simulink model "inertialDynamicsTestHarness"  (R2024a)
settings: configuration reference "standardSILConfiguraitonParams" (kept outside this file)
undefined symbols (not defined in the file): aircraftInitialEuler_rad, aircraftInitialPosInNED_m, aircraftInitialVelInBody_mps
settings Model: Creator=jerem  LastModifiedBy=jerem
settings ConfigSetRef: SourceName=standardSILConfiguraitonParams  SourceLocation=Base Workspace

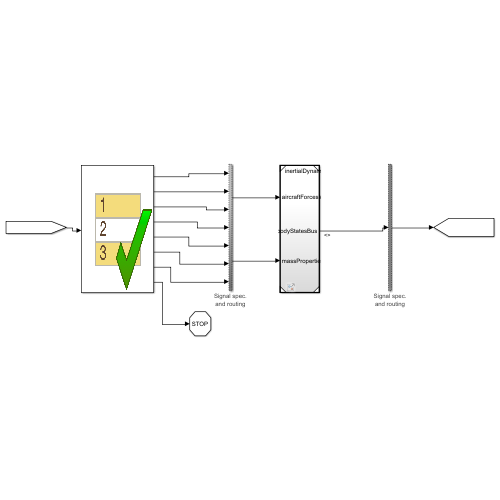
[thumbnail: Simulink's stored preview of the top-level diagram]
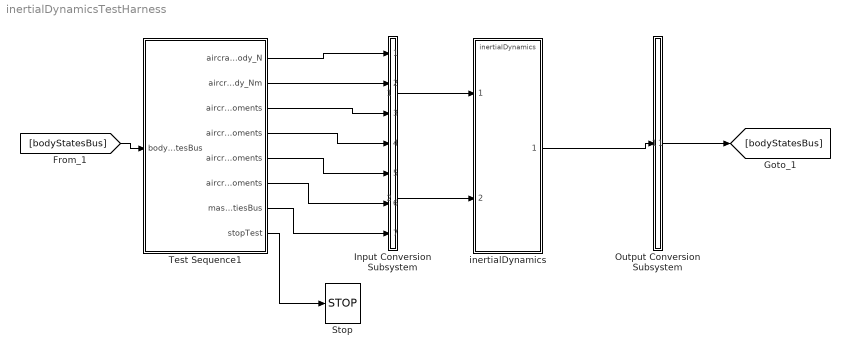
== system inertialDynamicsTestHarness ==
  Input Conversion Subsystem : Subsystem  Tag=__SLT_ICS__  Description=|
      | Signal spec.
      | and routing
      settings: AttributesFormatString=%<Description>
  Output Conversion Subsystem : Subsystem  Tag=__SLT_OCS__  Description=|
      | Signal spec.
      | and routing
      mask init:
      | ICDictionary = get_param(bdroot, 'DataDictionary');
      | if isempty(ICDictionary)
      |    ICScope = Simulink.data.BaseWorkspace;
      | else
      |    ICScope = Simulink.data.DataDictionary(ICDictionary);
      | end
      | 
      | IC1 = Simulink.Bus.createMATLABStruct('BodyStateBus', [], [1 1], ICScope);
      settings: AttributesFormatString=%<Description>
  Stop : Stop
  Test Sequence1 : Test Sequence  TreatAsAtomicUnit=on
  inertialDynamics : ModelReference  ModelNameDialog=inertialDynamics  SimulationMode=Normal  ModelReferenceVersion=1.34
  wires:
  Test Sequence1/1(aircraftForcesMomentsBus_forcesInBody_N) -> Input Conversion Subsystem/1(Inport_1)
  Test Sequence1/2(aircraftForcesMomentsBus_momentsInBody_Nm) -> Input Conversion Subsystem/2(Inport_2)
  Test Sequence1/3(aircraftForcesMomentsBus_aeroForcesMoments) -> Input Conversion Subsystem/3(Inport_3)
  Test Sequence1/4(aircraftForcesMomentsBus_engineForcesMoments) -> Input Conversion Subsystem/4(Inport_4)
  Test Sequence1/5(aircraftForcesMomentsBus_groundForcesMoments) -> Input Conversion Subsystem/5(Inport_5)
  Test Sequence1/6(aircraftForcesMomentsBus_weightForcesMoments) -> Input Conversion Subsystem/6(Inport_6)
  Test Sequence1/7(massPropertiesBus) -> Input Conversion Subsystem/7(Inport_7)
  [bodyStatesBus] -> Test Sequence1/1(bodyStatesBus)
  Output Conversion Subsystem/1(Outport_1) -> [bodyStatesBus]
  Test Sequence1/8(stopTest) -> Stop/1
  inertialDynamics/1 -> Output Conversion Subsystem/1(Inport_1)
  Input Conversion Subsystem/1(Outport_1) -> inertialDynamics/1
  Input Conversion Subsystem/2(Outport_2) -> inertialDynamics/2

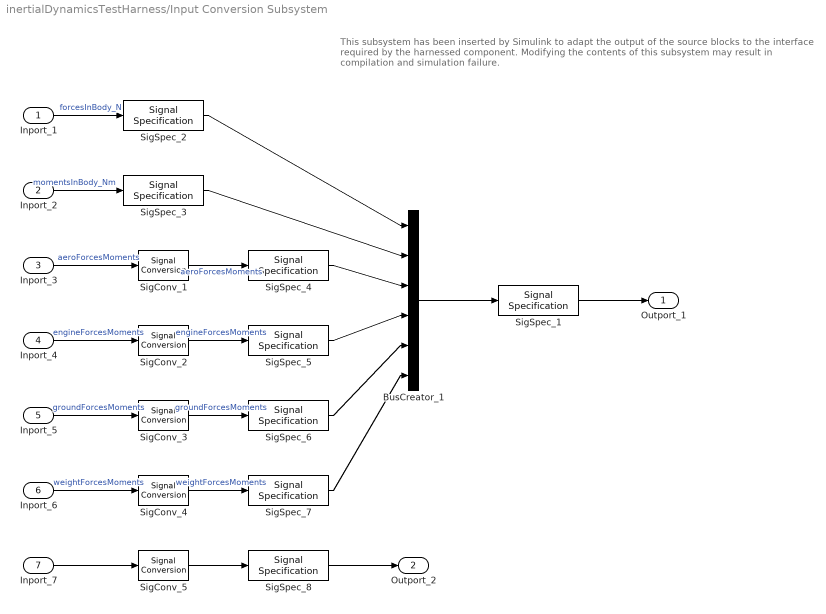
== system inertialDynamicsTestHarness/Input Conversion Subsystem ==
  note: This subsystem has been inserted by Simulink to adapt the output of the source blocks to the interface required by the harnessed component.
      |  Modifying the contents of this subsystem may result in compilation and simulation failure.
  Inport_1 : Inport
  Inport_2 : Inport  Port=2
  Inport_3 : Inport  Port=3
  Inport_4 : Inport  Port=4
  Inport_5 : Inport  Port=5
  Inport_6 : Inport  Port=6
  Inport_7 : Inport  Port=7
  BusCreator_1 : BusCreator  Inputs=6  OutDataTypeStr=Bus: AircraftForcesMomentsBus
  SigConv_{1..4} (4 alike) : SignalConversion  ConversionOutput=Nonvirtual bus  OverrideOpt=off
  SigConv_5 : SignalConversion  ConversionOutput=Virtual bus  OverrideOpt=off
  SigSpec_1 : SignalSpecification  OutDataTypeStr=Bus: AircraftForcesMomentsBus  SampleTime=[-1, 0]
  SigSpec_2 : SignalSpecification  OutDataTypeStr=double  Dimensions=[3]  SampleTime=[-1, 0]
  SigSpec_3 : SignalSpecification  OutDataTypeStr=double  Dimensions=[3]  SampleTime=[-1, 0]
  SigSpec_{4..7} (4 alike) : SignalSpecification  OutDataTypeStr=Bus: ComponentForcesMomentsBus  Dimensions=[1]  SampleTime=[-1, 0]  BusOutputAsStruct=on
  SigSpec_8 : SignalSpecification  OutDataTypeStr=Bus: MassPropertiesBus  SampleTime=[-1, 0]
  Outport_1 : Outport
  Outport_2 : Outport  Port=2
  wires:
  SigSpec_1/1 -> Outport_1/1
  BusCreator_1/1 -> SigSpec_1/1
  SigSpec_2/1 -> BusCreator_1/1
  Inport_1/1 -> SigSpec_2/1  "forcesInBody_N"
  SigSpec_3/1 -> BusCreator_1/2
  Inport_2/1 -> SigSpec_3/1  "momentsInBody_Nm"
  SigSpec_4/1 -> BusCreator_1/3
  SigConv_1/1 -> SigSpec_4/1  "aeroForcesMoments"
  Inport_3/1 -> SigConv_1/1  "aeroForcesMoments"
  SigSpec_5/1 -> BusCreator_1/4
  SigConv_2/1 -> SigSpec_5/1  "engineForcesMoments"
  Inport_4/1 -> SigConv_2/1  "engineForcesMoments"
  SigSpec_6/1 -> BusCreator_1/5
  SigConv_3/1 -> SigSpec_6/1  "groundForcesMoments"
  Inport_5/1 -> SigConv_3/1  "groundForcesMoments"
  SigSpec_7/1 -> BusCreator_1/6
  SigConv_4/1 -> SigSpec_7/1  "weightForcesMoments"
  Inport_6/1 -> SigConv_4/1  "weightForcesMoments"
  SigSpec_8/1 -> Outport_2/1
  SigConv_5/1 -> SigSpec_8/1
  Inport_7/1 -> SigConv_5/1

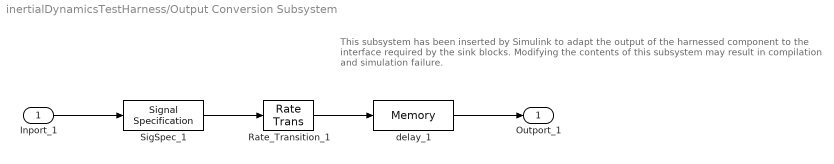
== system inertialDynamicsTestHarness/Output Conversion Subsystem ==
  note: This subsystem has been inserted by Simulink to adapt the output of the harnessed component to the interface required by the sink blocks.
      |  Modifying the contents of this subsystem may result in compilation and simulation failure.
  Inport_1 : Inport
  Rate_Transition_1 : RateTransition  OutPortSampleTimeOpt=Inherit
  SigSpec_1 : SignalSpecification  OutDataTypeStr=Bus: BodyStateBus  Dimensions=[1]
  delay_1 : Memory  InitialCondition=IC1
  Outport_1 : Outport
  wires:
  Inport_1/1 -> SigSpec_1/1
  SigSpec_1/1 -> Rate_Transition_1/1
  Rate_Transition_1/1 -> delay_1/1
  delay_1/1 -> Outport_1/1

== stateflow chart inertialDynamicsTestHarness/Test Sequence1 ==
  state Scenario_1
    state Initialize
      %% Initialize data outputs
      stopTest = false;
      aircraftForcesMomentsBus_forcesInBody_N = zeros(3, 1);
      aircraftForcesMomentsBus_momentsInBody_Nm = zeros(3, 1);
      aircraftForcesMomentsBus_aeroForcesMoments.forcesInBody_N = zeros(3,1);
      aircraftForcesMomentsBus_aeroForcesMoments.momentsInBody_Nm = zeros(3,1);
      aircraftForcesMomentsBus_engineForcesMoments.forcesInBody_N = zeros(3,1);
      aircraftForcesMomentsBus_engineForcesMoments.momentsInBody_Nm = zeros(3,1);
      aircraftForcesMomentsBus_groundForcesMoments.forcesInBody_N = zeros(3,1);
      aircraftForcesMomentsBus_groundForcesMoments.momentsInBody_Nm = zeros(3,1);
      aircraftForcesMomentsBus_weightForcesMoments.forcesInBody_N = zeros(3,1);
      aircraftForcesMomentsBus_weightForcesMoments.momentsInBody_Nm = zeros(3,1);
      massPropertiesBus.aircraftMass_kg = 0;
      massPropertiesBus.aircraftCg_m = zeros(3,1);
      massPropertiesBus.aircraftInertiaInBody_kgm2 = zeros(3,3);
      %% Initialize local parameters
      testForce = 1.0;
      %% Give aircraft mass and inertial to avoid divid by zero errors
      aircraftMass = 1.0;
      massPropertiesBus.aircraftMass_kg = aircraftMass;
      massPropertiesBus.aircraftInertiaInBody_kgm2 = eye(3,3);
    state Define_Test1_Inputs
      %% Apply non-zero forces
      aircraftForcesMomentsBus_forcesInBody_N = [testForce;0;0];
      aircraftForcesInNED_N = bodyStatesBus.DCM_be'*[testForce;0;0];
      apply_time = t(sec);
      interval_time = t(sec) - apply_time;
    state Test1
      % Test 1: verify position, velocity and accel match equations of motion
      % pos = 0.5*t^2*a + initPos
      % vel = 0.5*t^2*a + initVel
      % a = F/m
      verify(isClose(bodyStatesBus.aircraftPosInNED_m(1), 0.5*interval_time^2*aircraftForcesInNED_N(1)/aircraftMass + aircraftInitialPosInNED_m(1)))
      verify(isClose(bodyStatesBus.aircraftVelInBody_mps(1), interval_time*aircraftForcesMomentsBus_forcesInBody_N(1)/aircraftMass + aircraftInitialVelInBody_mps(1)))
      verify(isClose(bodyStatesBus.aircraftAccelInBody_mps2(1),aircraftForcesMomentsBus_forcesInBody_N(1)/aircraftMass))
      interval_time = t(sec) - apply_time;
    state EndTest
      stopTest = true;
    (default) -> Initialize
    Initialize -> Define_Test1_Inputs : [
        | true
        | ]
    Define_Test1_Inputs -> Test1 : [
        | true
        | ]
    Test1 -> EndTest : [
        | after(1,sec)
        | ]
  (default) -> Scenario_1 : {assert(Active_Scenario_Index == 1,'The value of Scenario Parameter ''Active_Scenario_Index'' is not valid. Use the index of the scenario to specify it.')}
  data: bodyStatesBus input Bus: BodyStateBus size=[1]; aircraftForcesMomentsBus_forcesInBody_N output double size=[3]; aircraftForcesMomentsBus_momentsInBody_Nm output double size=[3]; aircraftForcesMomentsBus_aeroForcesMoments output Bus: ComponentForcesMomentsBus size=[1]; aircraftForcesMomentsBus_engineForcesMoments output Bus: ComponentForcesMomentsBus size=[1]; aircraftForcesMomentsBus_groundForcesMoments output Bus: ComponentForcesMomentsBus size=[1]; aircraftForcesMomentsBus_weightForcesMoments output Bus: ComponentForcesMomentsBus size=[1]; massPropertiesBus output Bus: MassPropertiesBus size=[1]; interval_time local; aircraftInitialPosInNED_m parameter; aircraftInitialVelInBody_mps parameter; testForce local; aircraftMass local; Active_Scenario_Index parameter =1; apply_time local; aircraftInitialEuler_rad parameter; aircraftForcesInNED_N local; stopTest output
